simulink model "Question_4"  (R2024b)
settings: Solver=VariableStepAuto  StartTime=0.0  StopTime=10.0  RelTol=1e-3
model workspace (MAT data in the model file):
  L = 0.9939
  g = 9.8
  m = 10
settings Model: Creator=Sagar  LastModifiedBy=Sagar

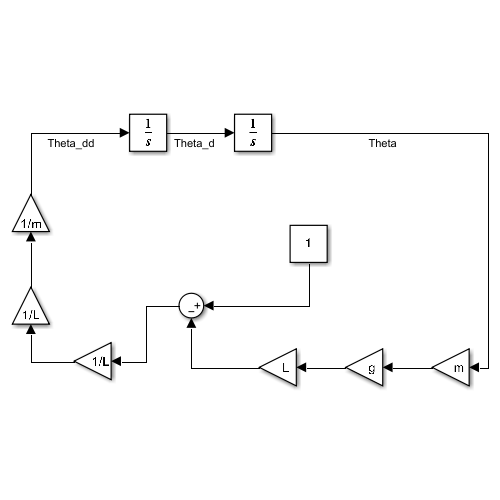
[thumbnail: Simulink's stored preview of the top-level diagram]
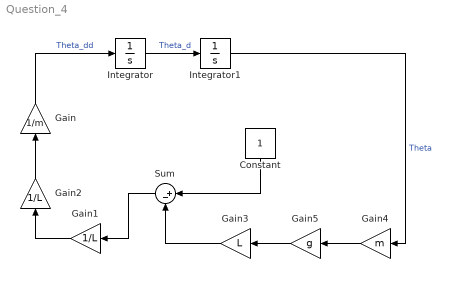
== system Question_4 ==
  Constant : Constant
  Gain : Gain  Gain=1/m
  Gain1 : Gain  Gain=1/L
  Gain2 : Gain  Gain=1/L
  Gain3 : Gain  Gain=L
  Gain4 : Gain  Gain=m
  Gain5 : Gain  Gain=g
  Integrator : Integrator
  Integrator1 : Integrator
  Sum : Sum  Inputs=|+-
  wires:
  Integrator/1 -> Integrator1/1  "Theta_d"
  Gain1/1 -> Gain2/1
  Gain2/1 -> Gain/1
  Gain/1 -> Integrator/1  "Theta_dd"
  Integrator1/1 -> Gain4/1  "Theta"
  Gain4/1 -> Gain5/1
  Gain5/1 -> Gain3/1
  Gain3/1 -> Sum/2
  Sum/1 -> Gain1/1
  Constant/1 -> Sum/1
